simulink model "CarSim_SCANeR_UDP_ACC_THESIS"  (R2019a)
settings: Solver=FixedStepAuto  StartTime=0.0  StopTime=inf  FixedStep=0.001  RelTol=1e-3  EnableMultiTasking=on
undefined symbols (not defined in the file or in its folder): DWORK0, DWORK1
libraries: simulink x14, xpcutilitieslib x2, xpcrtudplib x2, dspnetwork x1
(part 2 of 2)

== system CarSim_SCANeR_UDP_ACC_THESIS/ACC & CC1/LowerLevelController2_MASS_10% ==
  Ax_ref : Inport
  w : Inport  Port=2
  V_x : Inport  Port=3
  slope : Inport  Port=4
  Enable : Inport  Port=5
  APP : Inport  Port=6
  BPP_Act : Inport  Port=7
  SpaceControlEnable : Inport  Port=8
  GearRatio : Inport  Port=9
  LowerLevelController_sfcn : S-Function  FunctionName=LowerLevelController_sf  SFunctionModules=""  SFunctionDeploymentMode=off  EnableBusSupport=off  mask{rtw_sf_name=LowerLevelController_sf, showVar=off}
      mask prompts: rtw_sf_name "Simulink:masks:GenSFuncName_MP"; showVar "Simulink:masks:GenSFuncShowModuleList_MP"
      mask help: Simulink:masks:GenSFuncDesc_MD
      mask init: same as CarSim_SCANeR_UDP_ACC_THESIS/ACC & CC1/D_des1/D_des_sfcn
      settings: CopyFcn=|
      | if ~strcmp(get_param(gcb,'Linkstatus'),'none') && ...
      | ~strcmp(get_param(gcb,'Linkstatus'),'implicit')
      |   set_param(gcb,'LinkStatus','none');
      | end
      mask Help: eval('feval(''rtwprivate'',''rtwhelpview'',''rtw_sfcn_block'')');
      mask Display:
      | port_label('input',1,'Ax_ref');
      | port_label('input',2,'w');
      | port_label('input',3,'V_x');
      | port_label('input',4,'slope');
      | port_label('input',5,'Enable');
      | port_label('input',6,'APP');
      | port_label('input',7,'BPP_Act');
      | port_label('input',8,'SpaceControlEnable');
      | port_label('input',9,'GearRatio');
      | port_label('output',1,'EngineThrottle');
      | port_label('output',2,'BrakeForce');
  __InputSSForSFun__ : Subsystem
  __OutputSSForSFun__ : Subsystem
  EngineThrottle : Outport
  BrakeForce : Outport  Port=2
  wires:
  Ax_ref/1 -> __InputSSForSFun__/1(Ax_ref)
  w/1 -> __InputSSForSFun__/2(w)
  V_x/1 -> __InputSSForSFun__/3(V_x)
  slope/1 -> __InputSSForSFun__/4(slope)
  Enable/1 -> __InputSSForSFun__/5(Enable)
  APP/1 -> __InputSSForSFun__/6(APP)
  BPP_Act/1 -> __InputSSForSFun__/7(BPP_Act)
  SpaceControlEnable/1 -> __InputSSForSFun__/8(SpaceControlEnable)
  GearRatio/1 -> __InputSSForSFun__/9(GearRatio)
  __InputSSForSFun__/1(__UniqueOutportName__1__) -> LowerLevelController_sfcn/1
  __InputSSForSFun__/2(__UniqueOutportName__2__) -> LowerLevelController_sfcn/2
  __InputSSForSFun__/3(__UniqueOutportName__3__) -> LowerLevelController_sfcn/3
  __InputSSForSFun__/4(__UniqueOutportName__4__) -> LowerLevelController_sfcn/4
  __InputSSForSFun__/5(__UniqueOutportName__5__) -> LowerLevelController_sfcn/5
  __InputSSForSFun__/6(__UniqueOutportName__6__) -> LowerLevelController_sfcn/6
  __InputSSForSFun__/7(__UniqueOutportName__7__) -> LowerLevelController_sfcn/7
  __InputSSForSFun__/8(__UniqueOutportName__8__) -> LowerLevelController_sfcn/8
  __InputSSForSFun__/9(__UniqueOutportName__9__) -> LowerLevelController_sfcn/9
  LowerLevelController_sfcn/1 -> __OutputSSForSFun__/1(__UniqueInportName__1__)
  LowerLevelController_sfcn/2 -> __OutputSSForSFun__/2(__UniqueInportName__2__)
  __OutputSSForSFun__/1(EngineThrottle) -> EngineThrottle/1
  __OutputSSForSFun__/2(BrakeForce) -> BrakeForce/1

== system CarSim_SCANeR_UDP_ACC_THESIS/ACC & CC1/LowerLevelController2_ORGINAL ==
  Ax_ref : Inport
  w : Inport  Port=2
  V_x : Inport  Port=3
  slope : Inport  Port=4
  Enable : Inport  Port=5
  APP : Inport  Port=6
  BPP_Act : Inport  Port=7
  SpaceControlEnable : Inport  Port=8
  GearRatio : Inport  Port=9
  LowerLevelController_sfcn : S-Function  FunctionName=LowerLevelController_sf  SFunctionModules=""  SFunctionDeploymentMode=off  EnableBusSupport=off  mask{rtw_sf_name=LowerLevelController_sf, showVar=off}
      mask prompts: rtw_sf_name "Simulink:masks:GenSFuncName_MP"; showVar "Simulink:masks:GenSFuncShowModuleList_MP"
      mask help: Simulink:masks:GenSFuncDesc_MD
      mask init: same as CarSim_SCANeR_UDP_ACC_THESIS/ACC & CC1/D_des1/D_des_sfcn
      settings: CopyFcn=|
      | if ~strcmp(get_param(gcb,'Linkstatus'),'none') && ...
      | ~strcmp(get_param(gcb,'Linkstatus'),'implicit')
      |   set_param(gcb,'LinkStatus','none');
      | end
      mask Help: eval('feval(''rtwprivate'',''rtwhelpview'',''rtw_sfcn_block'')');
      mask Display:
      | port_label('input',1,'Ax_ref');
      | port_label('input',2,'w');
      | port_label('input',3,'V_x');
      | port_label('input',4,'slope');
      | port_label('input',5,'Enable');
      | port_label('input',6,'APP');
      | port_label('input',7,'BPP_Act');
      | port_label('input',8,'SpaceControlEnable');
      | port_label('input',9,'GearRatio');
      | port_label('output',1,'EngineThrottle');
      | port_label('output',2,'BrakeForce');
  __InputSSForSFun__ : Subsystem
  __OutputSSForSFun__ : Subsystem
  EngineThrottle : Outport
  BrakeForce : Outport  Port=2
  wires:
  __OutputSSForSFun__/2(BrakeForce) -> BrakeForce/1
  __OutputSSForSFun__/1(EngineThrottle) -> EngineThrottle/1
  LowerLevelController_sfcn/2 -> __OutputSSForSFun__/2(__UniqueInportName__2__)
  LowerLevelController_sfcn/1 -> __OutputSSForSFun__/1(__UniqueInportName__1__)
  __InputSSForSFun__/9(__UniqueOutportName__9__) -> LowerLevelController_sfcn/9
  __InputSSForSFun__/8(__UniqueOutportName__8__) -> LowerLevelController_sfcn/8
  __InputSSForSFun__/7(__UniqueOutportName__7__) -> LowerLevelController_sfcn/7
  __InputSSForSFun__/6(__UniqueOutportName__6__) -> LowerLevelController_sfcn/6
  __InputSSForSFun__/5(__UniqueOutportName__5__) -> LowerLevelController_sfcn/5
  __InputSSForSFun__/4(__UniqueOutportName__4__) -> LowerLevelController_sfcn/4
  __InputSSForSFun__/3(__UniqueOutportName__3__) -> LowerLevelController_sfcn/3
  __InputSSForSFun__/2(__UniqueOutportName__2__) -> LowerLevelController_sfcn/2
  __InputSSForSFun__/1(__UniqueOutportName__1__) -> LowerLevelController_sfcn/1
  GearRatio/1 -> __InputSSForSFun__/9(GearRatio)
  SpaceControlEnable/1 -> __InputSSForSFun__/8(SpaceControlEnable)
  BPP_Act/1 -> __InputSSForSFun__/7(BPP_Act)
  APP/1 -> __InputSSForSFun__/6(APP)
  Enable/1 -> __InputSSForSFun__/5(Enable)
  slope/1 -> __InputSSForSFun__/4(slope)
  V_x/1 -> __InputSSForSFun__/3(V_x)
  w/1 -> __InputSSForSFun__/2(w)
  Ax_ref/1 -> __InputSSForSFun__/1(Ax_ref)

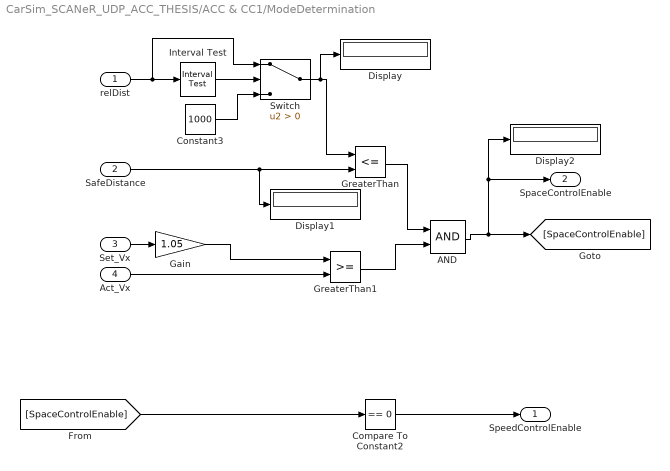
== system CarSim_SCANeR_UDP_ACC_THESIS/ACC & CC1/ModeDetermination ==
  relDist : Inport
  SafeDistance : Inport  Port=2
  Set_Vx : Inport  Port=3
  Act_Vx : Inport  Port=4
  AND : Logic  AllPortsSameDT=off  OutDataTypeStr=boolean
  Compare To Constant2 : simulink/Logic and Bit Operations/Compare To Constant  relop===  const=0  OutDataTypeStr=boolean
  Constant3 : Constant  Value=1000
  Display : Display
  Display1 : Display
  Display2 : Display
  Gain : Gain  Gain=1.05
  GreaterThan : RelationalOperator  Operator=<=  OutDataTypeStr=boolean  RndMeth=Simplest
  GreaterThan1 : RelationalOperator  OutDataTypeStr=boolean  RndMeth=Simplest
  Interval Test : simulink/Logic and Bit Operations/Interval Test  IntervalClosedRight=on  uplimit=150  IntervalClosedLeft=on  lowlimit=0.1  OutDataTypeStr=boolean
  Switch : Switch  Criteria=u2 > Threshold
  SpeedControlEnable : Outport
  SpaceControlEnable : Outport  Port=2
  wires:
  SafeDistance/1 -> Display1/1, GreaterThan/2
  Compare To Constant2/1 -> SpeedControlEnable/1
  AND/1 -> [SpaceControlEnable], Display2/1, SpaceControlEnable/1
  [SpaceControlEnable] -> Compare To Constant2/1
  Interval Test/1 -> Switch/2
  relDist/1 -> Interval Test/1, Switch/1
  Constant3/1 -> Switch/3
  Switch/1 -> Display/1, GreaterThan/1
  GreaterThan/1 -> AND/1
  Set_Vx/1 -> Gain/1
  Act_Vx/1 -> GreaterThan1/2
  Gain/1 -> GreaterThan1/1
  GreaterThan1/1 -> AND/2

== system CarSim_SCANeR_UDP_ACC_THESIS/ACC & CC1/ModeDetermination2 ==
  relDist : Inport
  SafeDistance : Inport  Port=2
  Set_Vx : Inport  Port=3
  Act_Vx : Inport  Port=4
  ModeDetermination_sfcn : S-Function  FunctionName=ModeDetermination_sf  SFunctionModules=""  SFunctionDeploymentMode=off  EnableBusSupport=off  mask{rtw_sf_name=ModeDetermination_sf, showVar=off}
      mask prompts: rtw_sf_name "Simulink:masks:GenSFuncName_MP"; showVar "Simulink:masks:GenSFuncShowModuleList_MP"
      mask help: Simulink:masks:GenSFuncDesc_MD
      mask init: same as CarSim_SCANeR_UDP_ACC_THESIS/ACC & CC1/D_des1/D_des_sfcn
      settings: CopyFcn=|
      | if ~strcmp(get_param(gcb,'Linkstatus'),'none') && ...
      | ~strcmp(get_param(gcb,'Linkstatus'),'implicit')
      |   set_param(gcb,'LinkStatus','none');
      | end
      mask Help: eval('feval(''rtwprivate'',''rtwhelpview'',''rtw_sfcn_block'')');
      mask Display:
      | port_label('input',1,'relDist');
      | port_label('input',2,'SafeDistance');
      | port_label('input',3,'Set_Vx');
      | port_label('input',4,'Act_Vx');
      | port_label('output',1,'SpeedControlEnable');
      | port_label('output',2,'SpaceControlEnable');
  __InputSSForSFun__ : Subsystem
  __OutputSSForSFun__ : Subsystem
  SpeedControlEnable : Outport
  SpaceControlEnable : Outport  Port=2
  wires:
  __OutputSSForSFun__/2(SpaceControlEnable) -> SpaceControlEnable/1
  __OutputSSForSFun__/1(SpeedControlEnable) -> SpeedControlEnable/1
  ModeDetermination_sfcn/2 -> __OutputSSForSFun__/2(__UniqueInportName__2__)
  ModeDetermination_sfcn/1 -> __OutputSSForSFun__/1(__UniqueInportName__1__)
  __InputSSForSFun__/4(__UniqueOutportName__4__) -> ModeDetermination_sfcn/4
  __InputSSForSFun__/3(__UniqueOutportName__3__) -> ModeDetermination_sfcn/3
  __InputSSForSFun__/2(__UniqueOutportName__2__) -> ModeDetermination_sfcn/2
  __InputSSForSFun__/1(__UniqueOutportName__1__) -> ModeDetermination_sfcn/1
  Act_Vx/1 -> __InputSSForSFun__/4(Act_Vx)
  Set_Vx/1 -> __InputSSForSFun__/3(Set_Vx)
  SafeDistance/1 -> __InputSSForSFun__/2(SafeDistance)
  relDist/1 -> __InputSSForSFun__/1(relDist)

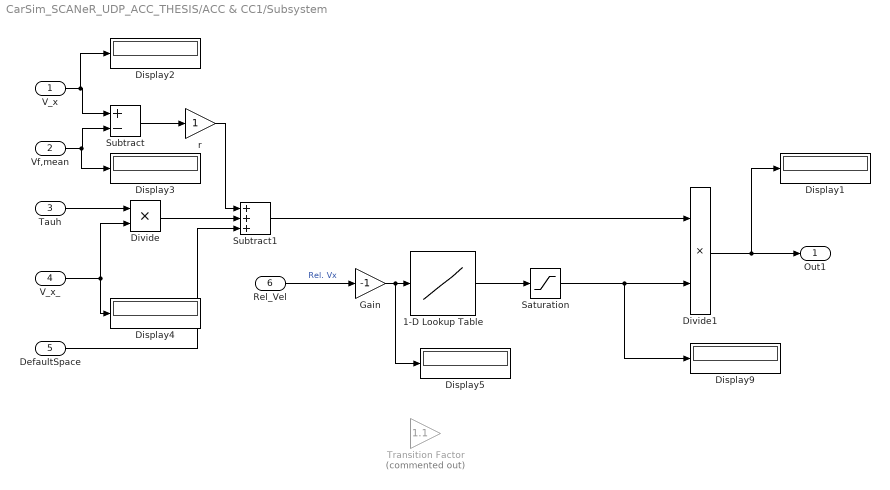
== system CarSim_SCANeR_UDP_ACC_THESIS/ACC & CC1/Subsystem ==
  V_x : Inport
  Vf,mean : Inport  Port=2
  Tauh : Inport  Port=3
  V_x_ : Inport  Port=4
  DefaultSpace : Inport  Port=5
  Rel_Vel : Inport  Port=6
  1-D Lookup Table : Lookup_n-D  NumberOfTableDimensions=1  BreakpointsForDimension1=[0,20]  Table=[1,1.1]  InternalRulePriority=Speed  RndMeth=Simplest  InputSameDT=on
  Display{1..5,9} (6 alike) : Display
  Divide : Product  Inputs=**
  Divide1 : Product  Inputs=**
  Gain : Gain  Gain=-1
  Saturation : Saturate  UpperLimit=1.50  LowerLimit=1.11
  Subtract : Sum  Inputs=+-
  Subtract1 : Sum  Inputs=+++
  Transition Factor : Gain  Commented=on  Gain=1.1
  r : Gain
  Out1 : Outport
  wires:
  Divide/1 -> Subtract1/2
  r/1 -> Subtract1/1
  Saturation/1 -> Divide1/2, Display9/1
  Subtract1/1 -> Divide1/1
  1-D Lookup Table/1 -> Saturation/1
  Subtract/1 -> r/1
  Gain/1 -> Display5/1, 1-D Lookup Table/1
  Rel_Vel/1 -> Gain/1  "Rel. Vx"
  DefaultSpace/1 -> Subtract1/3
  Divide1/1 -> Display1/1, Out1/1
  V_x/1 -> Display2/1, Subtract/1
  Tauh/1 -> Divide/1
  V_x_/1 -> Divide/2, Display4/1
  Vf,mean/1 -> Display3/1, Subtract/2

== system CarSim_SCANeR_UDP_ACC_THESIS/ACC & CC1/Subsystem1 ==
  SpeedControlEnable : Inport
  V_x : Inport  Port=2
  Vx_set : Inport  Port=3
  Enable : Inport  Port=4
  SpeedControlEnable_ : Inport  Port=5
  Display{,1..5} (6 alike) : Display
  Divide4 : Product  Inputs=***
  Logical Operator : Logic  AllPortsSameDT=off  OutDataTypeStr=boolean
  PID Controller2 : simulink/Continuous/PID Controller  Controller=PID  Form=Parallel  TimeDomain=Discrete-time  SampleTime=-1  IntegratorMethod=Forward Euler  FilterMethod=Forward Euler  ControllerParametersSource=internal  P=0.50  I=0.125  D=0  UseFilter=on  N=100  TunerSelectOption=Transfer Function Based (PID Tuner App)  InitialConditionSource=internal  InitialConditionForIntegrator=0  InitialConditionForFilter=0  DifferentiatorICPrevScaledInput=0  ExternalReset=rising  TrackingMode=off  Kt=1  LimitOutput=on  UpperSaturationLimit=inf  LowerSaturationLimit=-inf  LinearizeAsGain=on  AntiWindupMode=back-calculation  Kb=10  POutMin=[]  POutMax=[]  IOutMin=[]  IOutMax=[]  DOutMin=[]  DOutMax=[]  NOutMin=[]  NOutMax=[]  SumOutMin=[]  SumOutMax=[]  SaturationOutMin=[]  SaturationOutMax=[]  PParamMin=[]  PParamMax=[]  IParamMin=[]  IParamMax=[]  DParamMin=[]  DParamMax=[]  NParamMin=[]  NParamMax=[]  KbParamMin=[]  KbParamMax=[]  KtParamMin=[]  KtParamMax=[]  KbOutMin=[]  KbOutMax=[]  KtOutMin=[]  KtOutMax=[]  IntegratorOutMin=[]  IntegratorOutMax=[]  FilterOutMin=[]  FilterOutMax=[]  SumI1OutMin=[]  SumI1OutMax=[]  SumI2OutMin=[]  SumI2OutMax=[]  SumI3OutMin=[]  SumI3OutMax=[]  SumI4OutMin=[]  SumI4OutMax=[]  SumDOutMin=[]  SumDOutMax=[]  DifferentiatorOutMin=[]  DifferentiatorOutMax=[]  FilterDiffOutCoefMin=[]  FilterDiffOutCoefMax=[]  ReciprocalOutMin=[]  ReciprocalOutMax=[]  SumDenOutMin=[]  SumDenOutMax=[]  SumNumOutMin=[]  SumNumOutMax=[]  DivideOutMin=[]  DivideOutMax=[]  IntegratorContinuousStateAttributes=''  IntegratorStateMustResolveToSignalObject=off  IntegratorRTWStateStorageClass=Auto  FilterContinuousStateAttributes=''  FilterStateMustResolveToSignalObject=off  FilterRTWStateStorageClass=Auto  ParallelPVariant=InternalParameters  IdealPVariant=Disabled  IVariant=InternalParameters  DVariant=InternalParameters  IntegratorVariant=Discrete  SatVariant=Enabled  AWVariant=BackCalculation  PCopyVariant=Disabled  TRVariant=Disabled  FdbkBlocksVariant=Forward  IdealPFdbkVariant=Disabled  SatFdbkVariant=Disabled  DerivativeFilterVariant=ForwardEulerFilter  NVariant=InternalParameters  NCopyVariant=Disabled  FilterICVariant=InternalICsFilter  IntegratorICVariant=InternalICs  ExternalResetVariant=ExternalReset  TRSumVariant=Passthrough  SumFdbkVariant=Disabled  SumVariant=Sum_PID
      settings: LockScale=on
  Sum4 : Sum  Inputs=-+|
  PI_Ax : Outport
  wires:
  SpeedControlEnable/1 -> Display/1, Divide4/1
  [Enable] -> Display5/1, Divide4/3
  PID Controller2/1 -> Display4/1, Divide4/2  "Ax (ref)"
  Logical Operator/1 -> PID Controller2/2
  V_x/1 -> Display2/1, Sum4/1
  Enable/1 -> [Enable], Logical Operator/1
  Sum4/1 -> PID Controller2/1
  SpeedControlEnable_/1 -> Logical Operator/2
  Divide4/1 -> Display3/1, PI_Ax/1
  Vx_set/1 -> Display1/1, Sum4/2

== system CarSim_SCANeR_UDP_ACC_THESIS/ACC & CC1/Subsystem2 ==
  SpeedControlEnable : Inport
  V_x : Inport  Port=2
  Vx_set : Inport  Port=3
  Enable : Inport  Port=4
  SpeedControlEnable_ : Inport  Port=5
  Data Type Conversion : DataTypeConversion
  Data Type Conversion1 : DataTypeConversion
  Subsystem1_sfcn : S-Function  FunctionName=Subsystem1_sf  SFunctionModules=""  SFunctionDeploymentMode=off  EnableBusSupport=off  SFcnStateName=DWORK0,DWORK1  mask{rtw_sf_name=Subsystem1_sf, showVar=off}
      mask prompts: rtw_sf_name "Simulink:masks:GenSFuncName_MP"; showVar "Simulink:masks:GenSFuncShowModuleList_MP"
      mask help: Simulink:masks:GenSFuncDesc_MD
      mask init: same as CarSim_SCANeR_UDP_ACC_THESIS/ACC & CC1/D_des1/D_des_sfcn
      settings: SFcnIsStateOwnerBlock=on
      settings: CopyFcn=|
      | if ~strcmp(get_param(gcb,'Linkstatus'),'none') && ...
      | ~strcmp(get_param(gcb,'Linkstatus'),'implicit')
      |   set_param(gcb,'LinkStatus','none');
      | end
      mask Help: eval('feval(''rtwprivate'',''rtwhelpview'',''rtw_sfcn_block'')');
      mask Display:
      | port_label('input',1,'SpeedControlEnable');
      | port_label('input',2,'V_x');
      | port_label('input',3,'Vx_set');
      | port_label('input',4,'Enable');
      | port_label('input',5,'SpeedControlEnable_');
      | port_label('output',1,'PI_Ax');
  __InputSSForSFun__ : Subsystem
  __OutputSSForSFun__ : Subsystem
  PI_Ax : Outport
  wires:
  __OutputSSForSFun__/1(PI_Ax) -> PI_Ax/1
  Subsystem1_sfcn/1 -> __OutputSSForSFun__/1(__UniqueInportName__1__)
  __InputSSForSFun__/5(__UniqueOutportName__5__) -> Data Type Conversion1/1
  __InputSSForSFun__/4(__UniqueOutportName__4__) -> Subsystem1_sfcn/4
  __InputSSForSFun__/3(__UniqueOutportName__3__) -> Subsystem1_sfcn/3
  __InputSSForSFun__/2(__UniqueOutportName__2__) -> Subsystem1_sfcn/2
  __InputSSForSFun__/1(__UniqueOutportName__1__) -> Data Type Conversion/1
  SpeedControlEnable_/1 -> __InputSSForSFun__/5(SpeedControlEnable_)
  Enable/1 -> __InputSSForSFun__/4(Enable)
  Vx_set/1 -> __InputSSForSFun__/3(Vx_set)
  V_x/1 -> __InputSSForSFun__/2(V_x)
  SpeedControlEnable/1 -> __InputSSForSFun__/1(SpeedControlEnable)
  Data Type Conversion/1 -> Subsystem1_sfcn/1
  Data Type Conversion1/1 -> Subsystem1_sfcn/5

== system CarSim_SCANeR_UDP_ACC_THESIS/ACC & CC1/Subsystem3 ==
  State : Inport
  V_x : Inport  Port=2
  Ap : Inport  Port=3
  LeadAx : Inport  Port=4
  Enable : EnablePort
  Display{,1..3} (4 alike) : Display
  S-Function : S-Function  FunctionName=casadi_fun_acc  Parameters='acc.casadi', 'acc'  SFunctionDeploymentMode=off  EnableBusSupport=off
  Ax_des : Outport
  wires:
  State/1 -> S-Function/1, Display/1
  V_x/1 -> Display1/1, S-Function/2
  LeadAx/1 -> S-Function/4, Display2/1
  S-Function/1 -> Display3/1, Ax_des/1
  Ap/1 -> S-Function/3

== system CarSim_SCANeR_UDP_ACC_THESIS/ACC & CC1/Subsystem5 ==
  V_x : Inport
  Vf,mean : Inport  Port=2
  Tauh : Inport  Port=3
  V_x_ : Inport  Port=4
  DefaultSpace : Inport  Port=5
  Rel_Vel : Inport  Port=6
  Subsystem_sfcn : S-Function  FunctionName=Subsystem_sf  SFunctionModules=""  SFunctionDeploymentMode=off  EnableBusSupport=off  mask{rtw_sf_name=Subsystem_sf, showVar=off}
      mask prompts: rtw_sf_name "Simulink:masks:GenSFuncName_MP"; showVar "Simulink:masks:GenSFuncShowModuleList_MP"
      mask help: Simulink:masks:GenSFuncDesc_MD
      mask init: same as CarSim_SCANeR_UDP_ACC_THESIS/ACC & CC1/D_des1/D_des_sfcn
      settings: CopyFcn=|
      | if ~strcmp(get_param(gcb,'Linkstatus'),'none') && ...
      | ~strcmp(get_param(gcb,'Linkstatus'),'implicit')
      |   set_param(gcb,'LinkStatus','none');
      | end
      mask Help: eval('feval(''rtwprivate'',''rtwhelpview'',''rtw_sfcn_block'')');
      mask Display:
      | port_label('input',1,'V_x');
      | port_label('input',2,'Vf,mean');
      | port_label('input',3,'Tauh');
      | port_label('input',4,'V_x_');
      | port_label('input',5,'DefaultSpace');
      | port_label('input',6,'Rel_Vel');
      | port_label('output',1,'Out1');
  __InputSSForSFun__ : Subsystem
  __OutputSSForSFun__ : Subsystem
  Out1 : Outport
  wires:
  __OutputSSForSFun__/1(Out1) -> Out1/1
  Subsystem_sfcn/1 -> __OutputSSForSFun__/1(__UniqueInportName__1__)
  __InputSSForSFun__/6(__UniqueOutportName__6__) -> Subsystem_sfcn/6
  __InputSSForSFun__/5(__UniqueOutportName__5__) -> Subsystem_sfcn/5
  __InputSSForSFun__/4(__UniqueOutportName__4__) -> Subsystem_sfcn/4
  __InputSSForSFun__/3(__UniqueOutportName__3__) -> Subsystem_sfcn/3
  __InputSSForSFun__/2(__UniqueOutportName__2__) -> Subsystem_sfcn/2
  __InputSSForSFun__/1(__UniqueOutportName__1__) -> Subsystem_sfcn/1
  Rel_Vel/1 -> __InputSSForSFun__/6(Rel_Vel)
  DefaultSpace/1 -> __InputSSForSFun__/5(DefaultSpace)
  V_x_/1 -> __InputSSForSFun__/4(V_x_)
  Tauh/1 -> __InputSSForSFun__/3(Tauh)
  Vf,mean/1 -> __InputSSForSFun__/2(Vf,mean)
  V_x/1 -> __InputSSForSFun__/1(V_x)

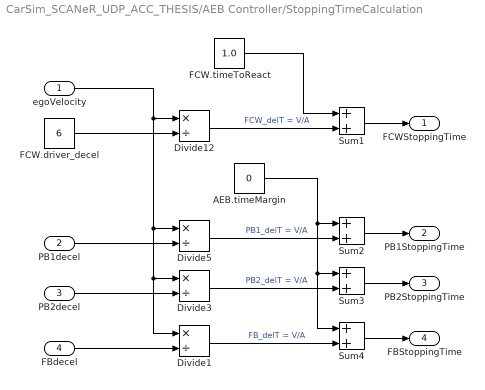
== system CarSim_SCANeR_UDP_ACC_THESIS/AEB Controller/StoppingTimeCalculation ==
  egoVelocity : Inport
  PB1decel : Inport  Port=2
  PB2decel : Inport  Port=3
  FBdecel : Inport  Port=4
  AEB.timeMargin : Constant  Value=0
  Divide{1,3,5,12} (4 alike) : Product  Inputs=*/
  FCW.driver_decel : Constant  Value=6
  FCW.timeToReact : Constant  Value=1.0
  Sum{1..4} (4 alike) : Sum
  FCWStoppingTime : Outport
  PB1StoppingTime : Outport  Port=2
  PB2StoppingTime : Outport  Port=3
  FBStoppingTime : Outport  Port=4
  wires:
  Divide12/1 -> Sum1/2  "FCW_delT = V/A"
  FCW.timeToReact/1 -> Sum1/1
  FBdecel/1 -> Divide1/2
  PB2decel/1 -> Divide3/2
  PB1decel/1 -> Divide5/2
  FCW.driver_decel/1 -> Divide12/2
  Divide1/1 -> Sum4/2  "FB_delT = V/A"
  Divide3/1 -> Sum3/2  "PB2_delT = V/A"
  Divide5/1 -> Sum2/2  "PB1_delT = V/A"
  egoVelocity/1 -> Divide12/1, Divide5/1, Divide3/1, Divide1/1
  AEB.timeMargin/1 -> Sum3/1, Sum4/1, Sum2/1
  Sum4/1 -> FBStoppingTime/1
  Sum3/1 -> PB2StoppingTime/1
  Sum2/1 -> PB1StoppingTime/1
  Sum1/1 -> FCWStoppingTime/1

== system CarSim_SCANeR_UDP_ACC_THESIS/AEB Controller/TTCCalculation ==
  mioDistance : Inport
  mioVelocity : Inport  Port=2
  AEB.headwayOffset : Constant  Value=0
  Abs : Abs
  Constant : Constant
  Divide11 : Product  Inputs=**
  Divide3 : Product  Inputs=*/
  Relational Operator : RelationalOperator  Operator=<  OutDataTypeStr=boolean  RndMeth=Simplest
  Saturation : Saturate  UpperLimit=100  LowerLimit=0.01
  Sign : Signum
  Sum : Sum  Inputs=+-
  const2 : Constant  Value=0.1  SampleTime=-1
  collision : Outport
  TTC : Outport  Port=2
  wires:
  Constant/1 -> Divide11/2
  Abs/1 -> Divide3/2  "mioVelSaturated"
  Divide11/1 -> TTC/1
  mioVelocity/1 -> Abs/1  "mioVelSaturated"
  Relational Operator/1 -> collision/1
  const2/1 -> Relational Operator/2
  Sum/1 -> Divide3/1, Relational Operator/1  "headway"
  AEB.headwayOffset/1 -> Sum/2
  Divide3/1 -> Divide11/1  "TTC"
  mioDistance/1 -> Sum/1  "mioDistance"

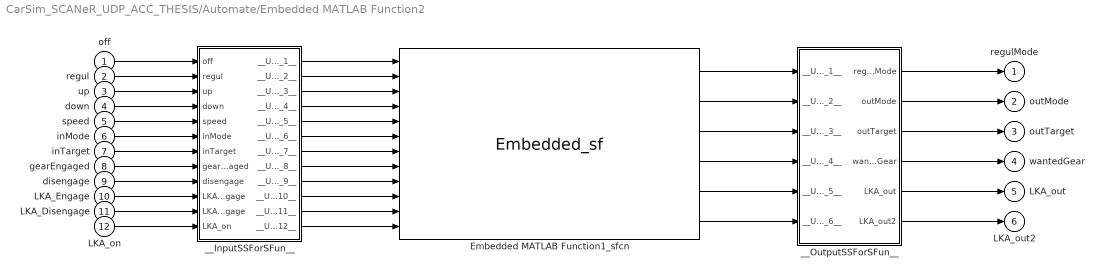
== system CarSim_SCANeR_UDP_ACC_THESIS/Automate/Embedded MATLAB Function2 ==
  off : Inport
  regul : Inport  Port=2
  up : Inport  Port=3
  down : Inport  Port=4
  speed : Inport  Port=5
  inMode : Inport  Port=6
  inTarget : Inport  Port=7
  gearEngaged : Inport  Port=8
  disengage : Inport  Port=9
  LKA_Engage : Inport  Port=10
  LKA_Disengage : Inport  Port=11
  LKA_on : Inport  Port=12
  Embedded MATLAB Function1_sfcn : S-Function  FunctionName=Embedded_sf  SFunctionModules=""  SFunctionDeploymentMode=off  EnableBusSupport=off  mask{rtw_sf_name=Embedded_sf, showVar=off}
      mask prompts: rtw_sf_name "Simulink:masks:GenSFuncName_MP"; showVar "Simulink:masks:GenSFuncShowModuleList_MP"
      mask help: Simulink:masks:GenSFuncDesc_MD
      mask init: same as CarSim_SCANeR_UDP_ACC_THESIS/ACC & CC1/D_des1/D_des_sfcn
      settings: CopyFcn=|
      | if ~strcmp(get_param(gcb,'Linkstatus'),'none') && ...
      | ~strcmp(get_param(gcb,'Linkstatus'),'implicit')
      |   set_param(gcb,'LinkStatus','none');
      | end
      mask Help: eval('feval(''rtwprivate'',''rtwhelpview'',''rtw_sfcn_block'')');
      mask Display:
      | port_label('input',1,'off');
      | port_label('input',2,'regul');
      | port_label('input',3,'up');
      | port_label('input',4,'down');
      | port_label('input',5,'speed');
      | port_label('input',6,'inMode');
      | port_label('input',7,'inTarget');
      | port_label('input',8,'gearEngaged');
      | port_label('input',9,'disengage');
      | port_label('input',10,'LKA_Engage');
      | port_label('input',11,'LKA_Disengage');
      | port_label('input',12,'LKA_on');
      | port_label('output',1,'regulMode');
      | port_label('output',2,'outMode');
      | port_label('output',3,'outTarget');
      | port_label('output',4,'wantedGear');
      | port_label('output',5,'LKA_out');
      | port_label('output',6,'LKA_out2');
  __InputSSForSFun__ : Subsystem
  __OutputSSForSFun__ : Subsystem
  regulMode : Outport
  outMode : Outport  Port=2
  outTarget : Outport  Port=3
  wantedGear : Outport  Port=4
  LKA_out : Outport  Port=5
  LKA_out2 : Outport  Port=6
  wires:
  __OutputSSForSFun__/6(LKA_out2) -> LKA_out2/1
  __OutputSSForSFun__/5(LKA_out) -> LKA_out/1
  __OutputSSForSFun__/4(wantedGear) -> wantedGear/1
  __OutputSSForSFun__/3(outTarget) -> outTarget/1
  __OutputSSForSFun__/2(outMode) -> outMode/1
  __OutputSSForSFun__/1(regulMode) -> regulMode/1
  Embedded MATLAB Function1_sfcn/6 -> __OutputSSForSFun__/6(__UniqueInportName__6__)
  Embedded MATLAB Function1_sfcn/5 -> __OutputSSForSFun__/5(__UniqueInportName__5__)
  Embedded MATLAB Function1_sfcn/4 -> __OutputSSForSFun__/4(__UniqueInportName__4__)
  Embedded MATLAB Function1_sfcn/3 -> __OutputSSForSFun__/3(__UniqueInportName__3__)
  Embedded MATLAB Function1_sfcn/2 -> __OutputSSForSFun__/2(__UniqueInportName__2__)
  Embedded MATLAB Function1_sfcn/1 -> __OutputSSForSFun__/1(__UniqueInportName__1__)
  __InputSSForSFun__/12(__UniqueOutportName__12__) -> Embedded MATLAB Function1_sfcn/12
  __InputSSForSFun__/11(__UniqueOutportName__11__) -> Embedded MATLAB Function1_sfcn/11
  __InputSSForSFun__/10(__UniqueOutportName__10__) -> Embedded MATLAB Function1_sfcn/10
  __InputSSForSFun__/9(__UniqueOutportName__9__) -> Embedded MATLAB Function1_sfcn/9
  __InputSSForSFun__/8(__UniqueOutportName__8__) -> Embedded MATLAB Function1_sfcn/8
  __InputSSForSFun__/7(__UniqueOutportName__7__) -> Embedded MATLAB Function1_sfcn/7
  __InputSSForSFun__/6(__UniqueOutportName__6__) -> Embedded MATLAB Function1_sfcn/6
  __InputSSForSFun__/5(__UniqueOutportName__5__) -> Embedded MATLAB Function1_sfcn/5
  __InputSSForSFun__/4(__UniqueOutportName__4__) -> Embedded MATLAB Function1_sfcn/4
  __InputSSForSFun__/3(__UniqueOutportName__3__) -> Embedded MATLAB Function1_sfcn/3
  __InputSSForSFun__/2(__UniqueOutportName__2__) -> Embedded MATLAB Function1_sfcn/2
  __InputSSForSFun__/1(__UniqueOutportName__1__) -> Embedded MATLAB Function1_sfcn/1
  LKA_on/1 -> __InputSSForSFun__/12(LKA_on)
  LKA_Disengage/1 -> __InputSSForSFun__/11(LKA_Disengage)
  LKA_Engage/1 -> __InputSSForSFun__/10(LKA_Engage)
  disengage/1 -> __InputSSForSFun__/9(disengage)
  gearEngaged/1 -> __InputSSForSFun__/8(gearEngaged)
  inTarget/1 -> __InputSSForSFun__/7(inTarget)
  inMode/1 -> __InputSSForSFun__/6(inMode)
  speed/1 -> __InputSSForSFun__/5(speed)
  down/1 -> __InputSSForSFun__/4(down)
  up/1 -> __InputSSForSFun__/3(up)
  regul/1 -> __InputSSForSFun__/2(regul)
  off/1 -> __InputSSForSFun__/1(off)

== system CarSim_SCANeR_UDP_ACC_THESIS/ACC & CC1/D_des1/__InputSSForSFun__ ==
  "Vf " : Inport
  reld : Inport  Port=2
  __UniqueOutportName__1__ : Outport
  __UniqueOutportName__2__ : Outport  Port=2
  wires:
  reld/1 -> __UniqueOutportName__2__/1
  "Vf "/1 -> __UniqueOutportName__1__/1

== system CarSim_SCANeR_UDP_ACC_THESIS/ACC & CC1/D_des1/__OutputSSForSFun__ ==
  __UniqueInportName__1__ : Inport
  deltad : Outport
  wires:
  __UniqueInportName__1__/1 -> deltad/1

== system CarSim_SCANeR_UDP_ACC_THESIS/ACC & CC1/LowerLevelController/WheelTorque ==
  A_x (m/s^2) : Inport
  V_x (m/s) : Inport  Port=2
  Slope (rad) : Inport  Port=3
  Add : Sum  Inputs=++++
  Cos : Trigonometry  Operator=cos
  Cos1 : Trigonometry
  Cr*M*g : Gain  Gain=(0.05)*1500*9.81
  M*g : Gain  Gain=(1500)*9.81
  M_eff : Gain  Gain=1.1*(1500)
  Rho*Cd*A : Gain  Gain=(1/2)*(1.2754)*(0.45)*1.5
  Rw (m) : Gain  Gain=0.20
  Square : Math  Operator=square  SaturateOnIntegerOverflow=on
  T_ref (N-m) : Outport  VectorParamsAs1DForOutWhenUnconnected=on
  wires:
  Rw (m)/1 -> T_ref (N-m)/1
  Add/1 -> Rw (m)/1
  M_eff/1 -> Add/4  "Inertial Force"
  A_x (m/s^2)/1 -> M_eff/1
  M*g/1 -> Add/3  "Slope Force"
  Cos1/1 -> M*g/1
  Cr*M*g/1 -> Add/2  "Rolling Resistance Force"
  Cos/1 -> Cr*M*g/1
  Slope (rad)/1 -> Cos/1, Cos1/1
  Rho*Cd*A/1 -> Add/1  "Aero Force"
  Square/1 -> Rho*Cd*A/1
  V_x (m/s)/1 -> Square/1

== system CarSim_SCANeR_UDP_ACC_THESIS/ACC & CC1/LowerLevelController2_MASS_10%/__InputSSForSFun__ ==
  Ax_ref : Inport
  w : Inport  Port=2
  V_x : Inport  Port=3
  slope : Inport  Port=4
  Enable : Inport  Port=5
  APP : Inport  Port=6
  BPP_Act : Inport  Port=7
  SpaceControlEnable : Inport  Port=8
  GearRatio : Inport  Port=9
  __UniqueOutportName__1__ : Outport
  __UniqueOutportName__2__ : Outport  Port=2
  __UniqueOutportName__3__ : Outport  Port=3
  __UniqueOutportName__4__ : Outport  Port=4
  __UniqueOutportName__5__ : Outport  Port=5
  __UniqueOutportName__6__ : Outport  Port=6
  __UniqueOutportName__7__ : Outport  Port=7
  __UniqueOutportName__8__ : Outport  Port=8
  __UniqueOutportName__9__ : Outport  Port=9
  wires:
  Ax_ref/1 -> __UniqueOutportName__1__/1
  w/1 -> __UniqueOutportName__2__/1
  V_x/1 -> __UniqueOutportName__3__/1
  slope/1 -> __UniqueOutportName__4__/1
  Enable/1 -> __UniqueOutportName__5__/1
  APP/1 -> __UniqueOutportName__6__/1
  BPP_Act/1 -> __UniqueOutportName__7__/1
  SpaceControlEnable/1 -> __UniqueOutportName__8__/1
  GearRatio/1 -> __UniqueOutportName__9__/1

== system CarSim_SCANeR_UDP_ACC_THESIS/ACC & CC1/LowerLevelController2_MASS_10%/__OutputSSForSFun__ ==
  __UniqueInportName__1__ : Inport
  __UniqueInportName__2__ : Inport  Port=2
  EngineThrottle : Outport
  BrakeForce : Outport  Port=2
  wires:
  __UniqueInportName__1__/1 -> EngineThrottle/1  "EngineThrottle"
  __UniqueInportName__2__/1 -> BrakeForce/1

== system CarSim_SCANeR_UDP_ACC_THESIS/ACC & CC1/LowerLevelController2_ORGINAL/__InputSSForSFun__ ==
  Ax_ref : Inport
  w : Inport  Port=2
  V_x : Inport  Port=3
  slope : Inport  Port=4
  Enable : Inport  Port=5
  APP : Inport  Port=6
  BPP_Act : Inport  Port=7
  SpaceControlEnable : Inport  Port=8
  GearRatio : Inport  Port=9
  __UniqueOutportName__1__ : Outport
  __UniqueOutportName__2__ : Outport  Port=2
  __UniqueOutportName__3__ : Outport  Port=3
  __UniqueOutportName__4__ : Outport  Port=4
  __UniqueOutportName__5__ : Outport  Port=5
  __UniqueOutportName__6__ : Outport  Port=6
  __UniqueOutportName__7__ : Outport  Port=7
  __UniqueOutportName__8__ : Outport  Port=8
  __UniqueOutportName__9__ : Outport  Port=9
  wires:
  GearRatio/1 -> __UniqueOutportName__9__/1
  SpaceControlEnable/1 -> __UniqueOutportName__8__/1
  BPP_Act/1 -> __UniqueOutportName__7__/1
  APP/1 -> __UniqueOutportName__6__/1
  Enable/1 -> __UniqueOutportName__5__/1
  slope/1 -> __UniqueOutportName__4__/1
  V_x/1 -> __UniqueOutportName__3__/1
  w/1 -> __UniqueOutportName__2__/1
  Ax_ref/1 -> __UniqueOutportName__1__/1

== system CarSim_SCANeR_UDP_ACC_THESIS/ACC & CC1/LowerLevelController2_ORGINAL/__OutputSSForSFun__ ==
  __UniqueInportName__1__ : Inport
  __UniqueInportName__2__ : Inport  Port=2
  EngineThrottle : Outport
  BrakeForce : Outport  Port=2
  wires:
  __UniqueInportName__2__/1 -> BrakeForce/1
  __UniqueInportName__1__/1 -> EngineThrottle/1  "EngineThrottle"

== system CarSim_SCANeR_UDP_ACC_THESIS/ACC & CC1/ModeDetermination2/__InputSSForSFun__ ==
  relDist : Inport
  SafeDistance : Inport  Port=2
  Set_Vx : Inport  Port=3
  Act_Vx : Inport  Port=4
  __UniqueOutportName__1__ : Outport
  __UniqueOutportName__2__ : Outport  Port=2
  __UniqueOutportName__3__ : Outport  Port=3
  __UniqueOutportName__4__ : Outport  Port=4
  wires:
  Act_Vx/1 -> __UniqueOutportName__4__/1
  Set_Vx/1 -> __UniqueOutportName__3__/1
  SafeDistance/1 -> __UniqueOutportName__2__/1
  relDist/1 -> __UniqueOutportName__1__/1

== system CarSim_SCANeR_UDP_ACC_THESIS/ACC & CC1/ModeDetermination2/__OutputSSForSFun__ ==
  __UniqueInportName__1__ : Inport
  __UniqueInportName__2__ : Inport  Port=2
  SpeedControlEnable : Outport
  SpaceControlEnable : Outport  Port=2
  wires:
  __UniqueInportName__2__/1 -> SpaceControlEnable/1
  __UniqueInportName__1__/1 -> SpeedControlEnable/1

== system CarSim_SCANeR_UDP_ACC_THESIS/ACC & CC1/Subsystem2/__InputSSForSFun__ ==
  SpeedControlEnable : Inport
  V_x : Inport  Port=2
  Vx_set : Inport  Port=3
  Enable : Inport  Port=4
  SpeedControlEnable_ : Inport  Port=5
  __UniqueOutportName__1__ : Outport
  __UniqueOutportName__2__ : Outport  Port=2
  __UniqueOutportName__3__ : Outport  Port=3
  __UniqueOutportName__4__ : Outport  Port=4
  __UniqueOutportName__5__ : Outport  Port=5
  wires:
  SpeedControlEnable_/1 -> __UniqueOutportName__5__/1
  Enable/1 -> __UniqueOutportName__4__/1
  Vx_set/1 -> __UniqueOutportName__3__/1
  V_x/1 -> __UniqueOutportName__2__/1
  SpeedControlEnable/1 -> __UniqueOutportName__1__/1

== system CarSim_SCANeR_UDP_ACC_THESIS/ACC & CC1/Subsystem2/__OutputSSForSFun__ ==
  __UniqueInportName__1__ : Inport
  PI_Ax : Outport
  wires:
  __UniqueInportName__1__/1 -> PI_Ax/1

== system CarSim_SCANeR_UDP_ACC_THESIS/ACC & CC1/Subsystem5/__InputSSForSFun__ ==
  V_x : Inport
  Vf,mean : Inport  Port=2
  Tauh : Inport  Port=3
  V_x_ : Inport  Port=4
  DefaultSpace : Inport  Port=5
  Rel_Vel : Inport  Port=6
  __UniqueOutportName__1__ : Outport
  __UniqueOutportName__2__ : Outport  Port=2
  __UniqueOutportName__3__ : Outport  Port=3
  __UniqueOutportName__4__ : Outport  Port=4
  __UniqueOutportName__5__ : Outport  Port=5
  __UniqueOutportName__6__ : Outport  Port=6
  wires:
  Rel_Vel/1 -> __UniqueOutportName__6__/1
  DefaultSpace/1 -> __UniqueOutportName__5__/1
  V_x_/1 -> __UniqueOutportName__4__/1
  Tauh/1 -> __UniqueOutportName__3__/1
  Vf,mean/1 -> __UniqueOutportName__2__/1
  V_x/1 -> __UniqueOutportName__1__/1

== system CarSim_SCANeR_UDP_ACC_THESIS/ACC & CC1/Subsystem5/__OutputSSForSFun__ ==
  __UniqueInportName__1__ : Inport
  Out1 : Outport
  wires:
  __UniqueInportName__1__/1 -> Out1/1

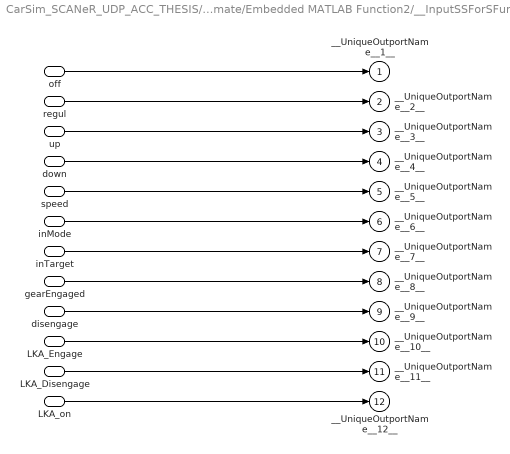
== system CarSim_SCANeR_UDP_ACC_THESIS/Automate/Embedded MATLAB Function2/__InputSSForSFun__ ==
  off : Inport
  regul : Inport  Port=2
  up : Inport  Port=3
  down : Inport  Port=4
  speed : Inport  Port=5
  inMode : Inport  Port=6
  inTarget : Inport  Port=7
  gearEngaged : Inport  Port=8
  disengage : Inport  Port=9
  LKA_Engage : Inport  Port=10
  LKA_Disengage : Inport  Port=11
  LKA_on : Inport  Port=12
  __UniqueOutportName__1__ : Outport
  __UniqueOutportName__2__ : Outport  Port=2
  __UniqueOutportName__3__ : Outport  Port=3
  __UniqueOutportName__4__ : Outport  Port=4
  __UniqueOutportName__5__ : Outport  Port=5
  __UniqueOutportName__6__ : Outport  Port=6
  __UniqueOutportName__7__ : Outport  Port=7
  __UniqueOutportName__8__ : Outport  Port=8
  __UniqueOutportName__9__ : Outport  Port=9
  __UniqueOutportName__10__ : Outport  Port=10
  __UniqueOutportName__11__ : Outport  Port=11
  __UniqueOutportName__12__ : Outport  Port=12
  wires:
  LKA_on/1 -> __UniqueOutportName__12__/1
  LKA_Disengage/1 -> __UniqueOutportName__11__/1
  LKA_Engage/1 -> __UniqueOutportName__10__/1
  disengage/1 -> __UniqueOutportName__9__/1
  gearEngaged/1 -> __UniqueOutportName__8__/1
  inTarget/1 -> __UniqueOutportName__7__/1
  inMode/1 -> __UniqueOutportName__6__/1
  speed/1 -> __UniqueOutportName__5__/1
  down/1 -> __UniqueOutportName__4__/1
  up/1 -> __UniqueOutportName__3__/1
  regul/1 -> __UniqueOutportName__2__/1
  off/1 -> __UniqueOutportName__1__/1

== system CarSim_SCANeR_UDP_ACC_THESIS/Automate/Embedded MATLAB Function2/__OutputSSForSFun__ ==
  __UniqueInportName__1__ : Inport
  __UniqueInportName__2__ : Inport  Port=2
  __UniqueInportName__3__ : Inport  Port=3
  __UniqueInportName__4__ : Inport  Port=4
  __UniqueInportName__5__ : Inport  Port=5
  __UniqueInportName__6__ : Inport  Port=6
  regulMode : Outport
  outMode : Outport  Port=2
  outTarget : Outport  Port=3
  wantedGear : Outport  Port=4
  LKA_out : Outport  Port=5
  LKA_out2 : Outport  Port=6
  wires:
  __UniqueInportName__6__/1 -> LKA_out2/1  "LKA_out2"
  __UniqueInportName__5__/1 -> LKA_out/1  "LKA_out"
  __UniqueInportName__4__/1 -> wantedGear/1  "wantedGear"
  __UniqueInportName__3__/1 -> outTarget/1  "outTarget"
  __UniqueInportName__2__/1 -> outMode/1  "outMode"
  __UniqueInportName__1__/1 -> regulMode/1  "regulMode"

== stateflow chart CarSim_SCANeR_UDP_ACC_THESIS/AEB Controller/AEB_Logic ==
  note: FCW/AEB Logic
  state Default
    entry: AEBstatus = 0;
    FCWactivate = 0;
    decel = 0;
  state FCW
    entry: AEBstatus = 0;
    FCWactivate = 1;
    decel = 0;
  state Partial_Braking1
    entry: AEBstatus = 1;
    FCWactivate = 1;
    decel = PB1decel;
  state Full_Braking
    entry: AEBstatus = 3;
    FCWactivate = 1;
    decel = FBdecel;
  state Partial_Braking2
    entry: AEBstatus = 2;
    FCWactivate = 1;
    decel = PB2decel;
  (default) -> Default
  Full_Braking -> Default : [stop==1]
  Partial_Braking1 -> Default [order 2] : [stop==1]
  Partial_Braking2 -> Default [order 2] : [stop==1]
  Default -> FCW : [(abs(TTC)<FCWtime)]
  FCW -> Default [order 2] : [abs(TTC)>=1.2*FCWtime]
  FCW -> Partial_Braking1 [order 1] : [(abs(TTC) < PB1time)]
  Partial_Braking1 -> Partial_Braking2 [order 1] : [(abs(TTC) < PB2time)]
  Partial_Braking2 -> Full_Braking [order 1] : [(abs(TTC) < FBtime)]
  data: FCWactivate output; TTC input; FCWtime input; PB1time input; PB2time input; FBtime input; PB1decel input; PB2decel input; FBdecel input; AEBstatus output; decel output; stop input

== matlab function CarSim_SCANeR_UDP_ACC_THESIS/Automate/Embedded MATLAB Function1 ==
  data: off input; regulMode output; regul input; up input; down input; speed input; inMode input; inTarget input; gearEngaged input; outMode output; outTarget output; disengage input; wantedGear output; LKA_Engage input; LKA_out output; LKA_Disengage input; LKA_out2 output; LKA_on input
function [regulMode, outMode, outTarget, wantedGear, LKA_out,LKA_out2] = fcn(off, regul, up, down, speed, inMode, inTarget,gearEngaged, disengage,LKA_Engage,LKA_Disengage,LKA_on)

ModeOff = 0;
ModeRegulOn = 1;
ModeRegulPause = 2;
minSpeed = 30;  %km/h
wantedGear = 0;

outMode = inMode;
outTarget = inTarget;

if ((regul == 1 && speed >= minSpeed) || (inMode == ModeRegulPause && (up == 1 || down == 1)))
    outMode = ModeRegulOn;
    outTarget = round(speed);
elseif inMode == ModeRegulPause && regul == 1
    outMode = ModeRegulOn;
elseif inMode == ModeRegulOn && (regul == 1 || disengage == 1)
    outMode = ModeRegulPause;
elseif inMode == ModeRegulOn && up == 1
    outTarget = inTarget + 1;
elseif inMode == ModeRegulOn && down == 1 && inTarget > minSpeed
    outTarget = inTarget - 1;
elseif off == 1
    outMode = ModeOff;
end

%Turn ACC on
if outMode == ModeRegulOn
    regulMode = 1;
    wantedGear = gearEngaged;
else
    regulMode = 0;
    wantedGear = 0;
end

%Turn LKA on

if (LKA_Engage == 1 && LKA_on == 1) || (LKA_Engage == 1 && LKA_on == 0);
    LKA_out = 1;
    LKA_out2 = 1;
elseif (LKA_Disengage == 1 && LKA_on == 1) || (LKA_Disengage == 1 && LKA_on == 0)
    LKA_out = 0;
    LKA_out2 = 0;
elseif (LKA_Engage == 0 && LKA_on == 1)
    LKA_out = 1;
    LKA_out2 = 1;
else
    LKA_out = 0;
    LKA_out2 = 0;
end
end
